simulink model "FOC_physical_2_Testing_mathmatical"  (R2024b)
settings: Solver=FixedStepAuto  StartTime=0.0  StopTime=4  FixedStep=1e-5  RelTol=1e-3
undefined symbols (not defined in the file): B, DiscIntNeverNeededParam, Down, dspblkCoreblockFVToolHelper, gcbh, GPTRIP1SEL, J, Ki_current, Ki_q, Ki_s, Ki_speed, Kp_current, Kp_q, Kp_s, Kp_speed, lambda, lamdaM, Ld, Ls, ma, P, Rs, T_max, T_period, Tc, TZ1, Up, Vdc
libraries: simulink x12, c2802xlib x7, spsIGBTDiodeLib x6, spsCurrentMeasurementLib x3, eeStairGenerator x2, spsStairGeneratorLib x2, spsDCVoltageSourceLib x1, spsPermanentMagnetSynchronousMachineLib x1, eeGeneralControl x1, mcbpositiondecoderlib x1, c280xlib x1, spspowerguiLib x1
(part 2 of 3)

== system FOC_physical_2_Testing_mathmatical/SVPWM Technique/Step 3- Determine the switching time of each transistor (S1 to S6)  ==
  T1 : Inport
  T2 : Inport  Port=2
  T0 : Inport  Port=3
  S : Inport  Port=4
  Fcn : Fcn  Expr=(T_period)-u(3)/2
  Fcn1 : Fcn  Expr=u(3)/2+u(2)
  Fcn2 : Fcn  Expr=u(3)/2
  Fcn3 : Fcn  Expr=u(3)/2+u(1)
  Mux1 : Mux  Inputs=3
  Sector detection1 : MATLAB Function  TreatAsAtomicUnit=on
  Ts1 : Outport
  Ts3 : Outport  Port=2
  Ts5 : Outport  Port=3
  wires:
  Sector detection1/1(Ts1) -> Ts1/1
  Sector detection1/3(Ts5) -> Ts5/1
  Sector detection1/2(Ts3) -> Ts3/1
  T0/1 -> Mux1/3
  T2/1 -> Mux1/2
  T1/1 -> Mux1/1
  Fcn2/1 -> Sector detection1/4(w)
  Fcn/1 -> Sector detection1/2(u)
  Fcn3/1 -> Sector detection1/5(g)
  Mux1/1 -> Fcn2/1, Fcn3/1, Fcn1/1, Fcn/1
  Fcn1/1 -> Sector detection1/3(v)
  S/1 -> Sector detection1/1(s)

== system FOC_physical_2_Testing_mathmatical/Subsystem/Forward Clacke ==
  Iu : Inport
  Iv : Inport  Port=2
  Iw : Inport  Port=3
  Gain : Gain  Gain=0.5
  Gain1 : Gain  Gain=0.5
  Gain2 : Gain  Gain=2/3
  Gain3 : Gain  Gain=sqrt(3)/2
  Gain4 : Gain  Gain=2/3
  Sum : Sum  Inputs=+--
  Sum1 : Sum  Inputs=+-
  I_alpha : Outport
  I_beta : Outport  Port=2
  wires:
  Iv/1 -> Gain/1, Sum1/1
  Gain/1 -> Sum/2
  Gain2/1 -> I_alpha/1
  Sum1/1 -> Gain3/1
  Gain1/1 -> Sum/3
  Iw/1 -> Gain1/1, Sum1/2
  Sum/1 -> Gain2/1
  Gain3/1 -> Gain4/1
  Iu/1 -> Sum/1
  Gain4/1 -> I_beta/1

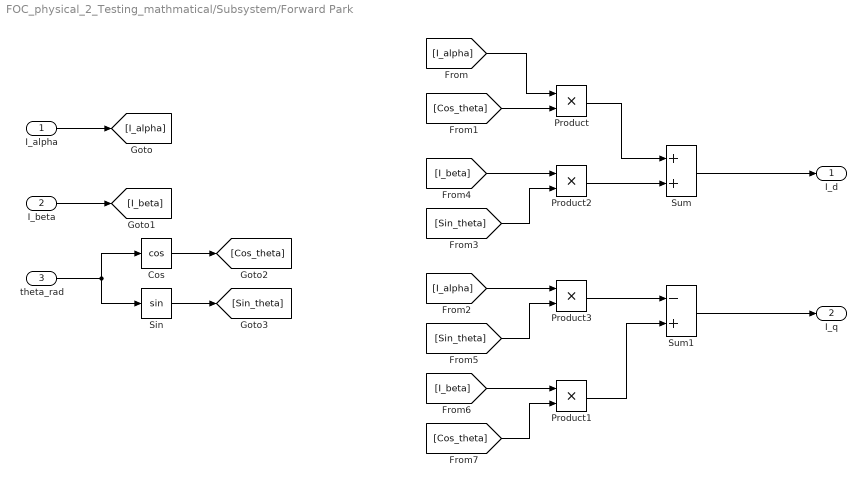
== system FOC_physical_2_Testing_mathmatical/Subsystem/Forward Park ==
  I_alpha : Inport
  I_beta : Inport  Port=2
  theta_rad : Inport  Port=3
  Cos : Trigonometry  Operator=cos
  Product{,1..3} (4 alike) : Product
  Sin : Trigonometry
  Sum : Sum
  Sum1 : Sum  Inputs=-+
  I_d : Outport
  I_q : Outport  Port=2
  wires:
  [Cos_theta] -> Product1/2
  [I_beta] -> Product1/1
  [Sin_theta] -> Product3/2
  [I_alpha] -> Product3/1
  Product1/1 -> Sum1/2
  [I_beta] -> Product2/1
  [Sin_theta] -> Product2/2
  [Cos_theta] -> Product/2
  Sin/1 -> [Sin_theta]
  Cos/1 -> [Cos_theta]
  theta_rad/1 -> Cos/1, Sin/1
  [I_alpha] -> Product/1
  I_beta/1 -> [I_beta]
  I_alpha/1 -> [I_alpha]
  Product3/1 -> Sum1/1
  Product2/1 -> Sum/2
  Product/1 -> Sum/1
  Sum1/1 -> I_q/1
  Sum/1 -> I_d/1

== system FOC_physical_2_Testing_mathmatical/Subsystem/Inverse Transformation ==
  Vq : Inport
  theta : Inport  Port=2
  Vd : Inport  Port=3
  "Inverse Park " : Subsystem  Commented=on
  dq to abc : Subsystem
  inverse Clark : Subsystem  Commented=on
  Va : Outport
  Vb : Outport  Port=2
  Vc : Outport  Port=3
  wires:
  theta/1 -> dq to abc/3(theta)
  Vq/1 -> dq to abc/1(V_q*)
  Vd/1 -> dq to abc/2(V_d*)
  dq to abc/1(Va*) -> Va/1
  dq to abc/2(Vb*) -> Vb/1
  dq to abc/3(Vc*) -> Vc/1

== system FOC_physical_2_Testing_mathmatical/Subsystem/SVPWM ==
  Va : Inport
  Vb : Inport  Port=2
  Vc : Inport  Port=3
  Vdc : Inport  Port=4
  Repeating Sequence : simulink/Sources/Repeating Sequence  rep_seq_t="[0 (T_period)/2  (T_period) ]"  rep_seq_y=[0 (T_period) 0]
  Scope : Scope  NumInputPorts=3
  Scope4 : Scope  NumInputPorts=4
  Sector detection : MATLAB Function  TreatAsAtomicUnit=on
  Subsystem : Subsystem
  Subsystem1 : Subsystem
  Subsystem2 : Subsystem
  Subsystem3 : Subsystem  Commented=on
  Subsystem4 : Subsystem  Commented=on
  Valpha and Vbeta Clark Trans : Subsystem
  TS1 : Outport
  TS3 : Outport  Port=2
  TS5 : Outport  Port=3
  wires:
  Valpha and Vbeta Clark Trans/1(Valpha) -> Subsystem/1(Valpha)
  Valpha and Vbeta Clark Trans/2(Vbeta) -> Subsystem/2(Vbeta)
  Vb/1 -> Scope/2, Valpha and Vbeta Clark Trans/2(Vb)
  Subsystem/2(angle) -> Sector detection/1(u), Subsystem1/2(angle)
  Vc/1 -> Scope/3, Valpha and Vbeta Clark Trans/3(Vc)
  Va/1 -> Valpha and Vbeta Clark Trans/1(Va), Scope/1
  Subsystem/1(Vref) -> Subsystem1/1(Vref)
  Sector detection/1(S) -> Subsystem1/3(Sector), Subsystem2/4(Sector definiton)  "Sector definiton"
  Subsystem1/2(T2) -> Scope4/2, Subsystem2/2(T2)
  Subsystem1/1(T1) -> Scope4/1, Subsystem2/1(T1)
  Subsystem1/3(T0) -> Subsystem2/3(T0), Scope4/3
  Subsystem2/2(TS3) -> TS3/1
  Subsystem2/1(TS1) -> TS1/1
  Subsystem2/3(TS5) -> TS5/1
  Vdc/1 -> Subsystem1/4(Vdc)

== system FOC_physical_2_Testing_mathmatical/Subsystem/Speed PI Controller with anti-windup ==
  Mech Speed ref : Inport
  Speed act : Inport  Port=2
  " max current" : Saturate  UpperLimit=T_max/((3/2)*lamdaM*P)  LowerLimit=0
  Abs : Abs  SaturateOnIntegerOverflow=off
  Abs1 : Abs  SaturateOnIntegerOverflow=off
  Compare To Constant1 : simulink/Logic and Bit Operations/Compare To Constant  relop=<=  const=1e-4  OutDataTypeStr=boolean
  Integrator2 : Integrator  ExternalReset=falling
  "Ki " : Gain  Gain=Ki_speed
  Kp : Gain  Gain=Kp_speed
  Product : Product  Inputs=3
  Scope : Scope
  Scope1 : Scope  NumInputPorts=2
  Scope2 : Scope  NumInputPorts=2
  Scope3 : Scope  NumInputPorts=3
  Scope4 : Scope  NumInputPorts=2
  Sum : Sum  Inputs=|+-
  Sum1 : Sum
  Sum2 : Sum  Inputs=|-+
  rpm_to_rad/s : Gain  Gain=pi/30
  stop integration at low speed : Relay  OnSwitchValue=100  OffSwitchValue=-100
  I_q* : Outport
  wires:
  " max current"/1 -> Scope2/1, Sum2/1, I_q*/1
  Sum/1 -> rpm_to_rad/s/1
  rpm_to_rad/s/1 -> Kp/1, Scope3/1, "Ki "/1
  stop integration at low speed/1 -> Integrator2/2, Product/3, Scope4/1
  Abs1/1 -> Scope4/2, stop integration at low speed/1
  Compare To Constant1/1 -> Scope/1, Product/1
  Abs/1 -> Compare To Constant1/1
  Sum2/1 -> Abs/1
  Sum1/1 -> " max current"/1, Sum2/2, Scope3/3, Scope2/2
  Integrator2/1 -> Sum1/2, Scope1/2
  Product/1 -> Integrator2/1, Scope1/1
  "Ki "/1 -> Product/2
  Kp/1 -> Sum1/1, Scope3/2
  Speed act/1 -> Sum/2, Abs1/1
  Mech Speed ref/1 -> Sum/1

== system FOC_physical_2_Testing_mathmatical/Subsystem/Subsystem ==
  Va : Inport
  Vb : Inport  Port=2
  Vc : Inport  Port=3
  TL : Inport  Port=4
  Current Calculation1 : Subsystem
  Display : Display
  Display1 : Display
  Display2 : Display
  Gain2 : Gain  Gain=60/(2*pi)
  Gain3 : Gain  Gain=1/P
  Park and Clark transformation1 : Subsystem
  Scope : Scope  NumInputPorts=2
  Speed1 : Subsystem
  Torque 1 : Subsystem
  Te : Outport
  Wm : Outport  Port=2
  Id : Outport  Port=3
  Iq : Outport  Port=4
  Theta : Outport  Port=5
  wires:
  [Wr] -> Current Calculation1/3(wr)
  Va/1 -> Display2/1, Park and Clark transformation1/1(Va)
  Park and Clark transformation1/2(Vq) -> Current Calculation1/2(Vq), Display1/1
  Torque 1/1(Te) -> Scope/2, Te/1, Speed1/1(Te)
  Speed1/1(wr) -> Gain2/1, [Wr]
  Park and Clark transformation1/1(Vd) -> Display/1, Current Calculation1/1(Vd)
  Gain2/1 -> Gain3/1
  Speed1/2(Theta) -> Park and Clark transformation1/4(Theta), Theta/1
  Current Calculation1/2(Iq) -> Torque 1/2(Iq), Iq/1
  Current Calculation1/1(Id) -> Id/1, Torque 1/1(Id)
  Vb/1 -> Park and Clark transformation1/2(Vb)
  Gain3/1 -> Scope/1, Wm/1  "N_actual"
  Vc/1 -> Park and Clark transformation1/3(Vc)
  TL/1 -> Speed1/2(TL)

== system FOC_physical_2_Testing_mathmatical/Subsystem/Voltage Decoupling  ==
  V_q* : Inport
  V_d* : Inport  Port=2
  Gain : Gain  Gain=2*pi/60
  Gain1 : Gain  Gain=P
  Gain2 : Gain  Gain=P
  Gain3 : Gain  Gain=P
  Gain4 : Gain  Gain=2*pi/60
  Gain5 : Gain  Gain=2*pi/60
  Lambda_m : Constant  Value=lamdaM
  Lambda_m1 : Constant  Value=Ls
  Ld : Constant  Value=Ls
  Product : Product  Inputs=3
  Product1 : Product
  Product2 : Product  Inputs=3
  Sum3 : Sum  Inputs=+++
  Sum4 : Sum  Inputs=|+-
  Vq : Outport
  Vd : Outport  Port=2
  wires:
  [Id] -> Product/1
  V_q*/1 -> Sum3/2
  Gain1/1 -> Product2/2
  Product2/1 -> Sum4/2
  [Iq] -> Product2/1
  Product1/1 -> Sum3/3
  [W_act] -> Gain5/1
  Gain2/1 -> Product/2
  [W_act] -> Gain/1
  Ld/1 -> Product/3
  [W_act] -> Gain4/1
  Product/1 -> Sum3/1
  Gain3/1 -> Product1/1
  Lambda_m/1 -> Product1/2
  Lambda_m1/1 -> Product2/3
  Sum3/1 -> Vq/1
  V_d*/1 -> Sum4/1
  Sum4/1 -> Vd/1
  Gain/1 -> Gain2/1
  Gain4/1 -> Gain3/1
  Gain5/1 -> Gain1/1

== system FOC_physical_2_Testing_mathmatical/Subsystem/d-current PI controller with anti-windup ==
  Id command : Inport
  Id act : Inport  Port=2
  Integrator2 : Integrator
  "Ki " : Gain  Gain=Ki_current
  Kp : Gain  Gain=Kp_current
  Product : Product
  Scope : Scope
  Scope1 : Scope  NumInputPorts=2
  Scope2 : Scope  NumInputPorts=2
  Scope3 : Scope  NumInputPorts=3
  Sum : Sum  Inputs=|+-
  Sum1 : Sum
  V_d* : Outport
  wires:
  Sum1/1 -> V_d*/1, Scope3/3, Scope2/2
  Integrator2/1 -> Sum1/2, Scope1/2
  Product/1 -> Integrator2/1, Scope1/1
  "Ki "/1 -> Product/2
  Kp/1 -> Sum1/1, Scope3/2
  Sum/1 -> Kp/1, Scope3/1, "Ki "/1
  Id act/1 -> Sum/2
  Id command/1 -> Sum/1
  [stop_d_integrator] -> Product/1, Scope/1

== system FOC_physical_2_Testing_mathmatical/Subsystem/q-current PI controller with anti-windup ==
  Iq command : Inport
  Iq act : Inport  Port=2
  Integrator2 : Integrator
  "Ki " : Gain  Gain=Ki_current
  Kp : Gain  Gain=Kp_current
  Product : Product
  Scope : Scope
  Scope1 : Scope  NumInputPorts=2
  Scope2 : Scope  NumInputPorts=2
  Scope3 : Scope  NumInputPorts=3
  Sum : Sum  Inputs=|+-
  Sum1 : Sum
  V_q* : Outport
  wires:
  Iq command/1 -> Sum/1
  Iq act/1 -> Sum/2
  Sum/1 -> "Ki "/1, Scope3/1, Kp/1
  Kp/1 -> Scope3/2, Sum1/1
  "Ki "/1 -> Product/2
  Product/1 -> Integrator2/1, Scope1/1
  Integrator2/1 -> Scope1/2, Sum1/2
  Sum1/1 -> V_q*/1, Scope2/2, Scope3/3
  [stop_q_integrator] -> Scope/1, Product/1

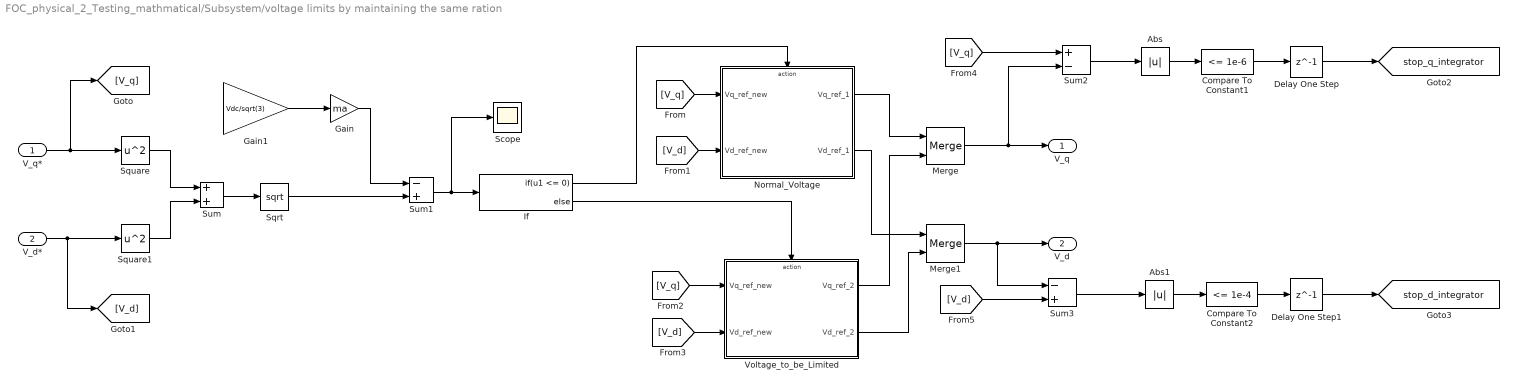
== system FOC_physical_2_Testing_mathmatical/Subsystem/voltage limits by maintaining the same ration ==
  V_q* : Inport
  V_d* : Inport  Port=2
  Abs : Abs  SaturateOnIntegerOverflow=off
  Abs1 : Abs  SaturateOnIntegerOverflow=off
  Compare To Constant1 : simulink/Logic and Bit Operations/Compare To Constant  relop=<=  const=1e-6  OutDataTypeStr=boolean
  Compare To Constant2 : simulink/Logic and Bit Operations/Compare To Constant  relop=<=  const=1e-4  OutDataTypeStr=boolean
  Delay One Step : Delay  DelayLength=1
  Delay One Step1 : Delay  DelayLength=1
  Gain : Gain  Gain=ma
  Gain1 : Gain  Gain=Vdc/sqrt(3)
  If : If  IfExpression=u1 <= 0
  Merge : Merge
  Merge1 : Merge
  Normal_Voltage : Subsystem  TreatAsAtomicUnit=on
      settings: RTWSystemCode=Inline  RTWFcnNameOpts=Use subsystem name  RTWFileNameOpts=Use subsystem name
  Scope : Scope
  Sqrt : Sqrt
  Square : Math  Operator=square
  Square1 : Math  Operator=square
  Sum : Sum
  Sum1 : Sum  Inputs=-+
  Sum2 : Sum  Inputs=+-
  Sum3 : Sum  Inputs=-+
  Voltage_to_be_Limited : Subsystem  TreatAsAtomicUnit=on
      settings: RTWSystemCode=Inline  RTWFcnNameOpts=Use subsystem name  RTWFileNameOpts=Use subsystem name
  V_q : Outport
  V_d : Outport  Port=2
  tag scope: stop_d_integrator=global, stop_q_integrator=global
  wires:
  V_q*/1 -> [V_q], Square/1
  V_d*/1 -> [V_d], Square1/1
  Sum/1 -> Sqrt/1
  Square/1 -> Sum/1
  Square1/1 -> Sum/2
  Sqrt/1 -> Sum1/2
  Merge/1 -> Sum2/2, V_q/1
  Gain/1 -> Sum1/1
  Sum1/1 -> Scope/1, If/1
  If/1 -> Normal_Voltage/Action
  [V_q] -> Normal_Voltage/1(Vq_ref_new)
  [V_d] -> Normal_Voltage/2(Vd_ref_new)
  If/2 -> Voltage_to_be_Limited/Action
  Voltage_to_be_Limited/1(Vq_ref_2) -> Merge/2
  Normal_Voltage/1(Vq_ref_1) -> Merge/1
  Voltage_to_be_Limited/2(Vd_ref_2) -> Merge1/2
  Normal_Voltage/2(Vd_ref_1) -> Merge1/1
  [V_q] -> Voltage_to_be_Limited/1(Vq_ref_new)
  [V_d] -> Voltage_to_be_Limited/2(Vd_ref_new)
  [V_q] -> Sum2/1
  Merge1/1 -> Sum3/1, V_d/1
  [V_d] -> Sum3/2
  Delay One Step/1 -> [stop_q_integrator]
  Delay One Step1/1 -> [stop_d_integrator]
  Abs/1 -> Compare To Constant1/1
  Compare To Constant1/1 -> Delay One Step/1
  Sum2/1 -> Abs/1
  Sum3/1 -> Abs1/1
  Abs1/1 -> Compare To Constant2/1
  Compare To Constant2/1 -> Delay One Step1/1
  Gain1/1 -> Gain/1

== system FOC_physical_2_Testing_mathmatical/Subsystem3/Forward Clacke ==
  Iu : Inport
  Iv : Inport  Port=2
  Iw : Inport  Port=3
  Gain : Gain  Gain=0.5
  Gain1 : Gain  Gain=0.5
  Gain2 : Gain  Gain=2/3
  Gain3 : Gain  Gain=sqrt(3)/2
  Gain4 : Gain  Gain=2/3
  Sum : Sum  Inputs=+--
  Sum1 : Sum  Inputs=+-
  I_alpha : Outport
  I_beta : Outport  Port=2
  wires:
  Iv/1 -> Gain/1, Sum1/1
  Gain/1 -> Sum/2
  Gain2/1 -> I_alpha/1
  Sum1/1 -> Gain3/1
  Gain1/1 -> Sum/3
  Iw/1 -> Gain1/1, Sum1/2
  Sum/1 -> Gain2/1
  Gain3/1 -> Gain4/1
  Iu/1 -> Sum/1
  Gain4/1 -> I_beta/1

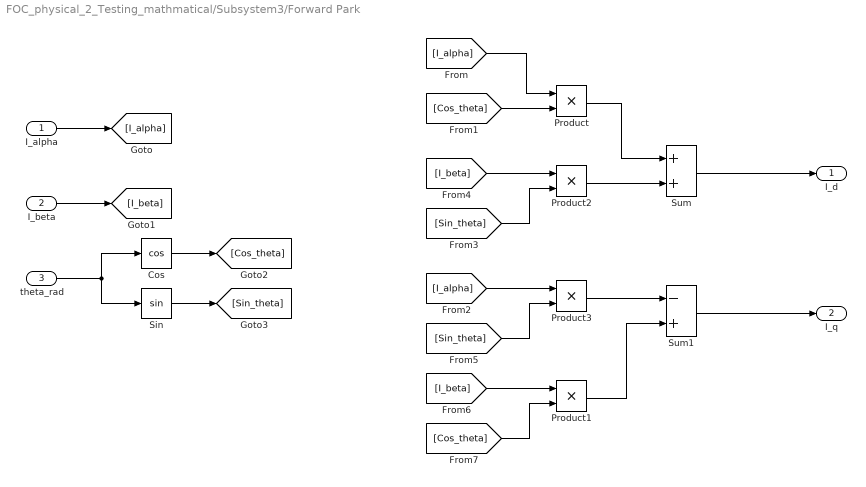
== system FOC_physical_2_Testing_mathmatical/Subsystem3/Forward Park ==
  I_alpha : Inport
  I_beta : Inport  Port=2
  theta_rad : Inport  Port=3
  Cos : Trigonometry  Operator=cos
  Product{,1..3} (4 alike) : Product
  Sin : Trigonometry
  Sum : Sum
  Sum1 : Sum  Inputs=-+
  I_d : Outport
  I_q : Outport  Port=2
  wires:
  [Cos_theta] -> Product1/2
  [I_beta] -> Product1/1
  [Sin_theta] -> Product3/2
  [I_alpha] -> Product3/1
  Product1/1 -> Sum1/2
  [I_beta] -> Product2/1
  [Sin_theta] -> Product2/2
  [Cos_theta] -> Product/2
  Sin/1 -> [Sin_theta]
  Cos/1 -> [Cos_theta]
  theta_rad/1 -> Cos/1, Sin/1
  [I_alpha] -> Product/1
  I_beta/1 -> [I_beta]
  I_alpha/1 -> [I_alpha]
  Product3/1 -> Sum1/1
  Product2/1 -> Sum/2
  Product/1 -> Sum/1
  Sum1/1 -> I_q/1
  Sum/1 -> I_d/1

== system FOC_physical_2_Testing_mathmatical/Subsystem3/Inverse Transformation ==
  Vq : Inport
  theta : Inport  Port=2
  Vd : Inport  Port=3
  "Inverse Park " : Subsystem  Commented=on
  dq to abc : Subsystem
  inverse Clark : Subsystem  Commented=on
  Va : Outport
  Vb : Outport  Port=2
  Vc : Outport  Port=3
  wires:
  theta/1 -> dq to abc/3(theta)
  Vq/1 -> dq to abc/1(V_q*)
  Vd/1 -> dq to abc/2(V_d*)
  dq to abc/1(Va*) -> Va/1
  dq to abc/2(Vb*) -> Vb/1
  dq to abc/3(Vc*) -> Vc/1

== system FOC_physical_2_Testing_mathmatical/Subsystem3/SVPWM ==
  Va : Inport
  Vb : Inport  Port=2
  Vc : Inport  Port=3
  Vdc : Inport  Port=4
  Scope : Scope  NumInputPorts=3
  Scope4 : Scope  NumInputPorts=4
  Sector detection : MATLAB Function  TreatAsAtomicUnit=on
  Subsystem : Subsystem
  Subsystem1 : Subsystem
  Subsystem2 : Subsystem
  Subsystem3 : Subsystem  Commented=on
  Subsystem4 : Subsystem  Commented=on
  Valpha and Vbeta Clark Trans : Subsystem
  TS1 : Outport
  TS3 : Outport  Port=2
  TS5 : Outport  Port=3
  wires:
  Valpha and Vbeta Clark Trans/1(Valpha) -> Subsystem/1(Valpha)
  Valpha and Vbeta Clark Trans/2(Vbeta) -> Subsystem/2(Vbeta)
  Vb/1 -> Scope/2, Valpha and Vbeta Clark Trans/2(Vb)
  Subsystem/2(angle) -> Sector detection/1(u), Subsystem1/2(angle)
  Vc/1 -> Scope/3, Valpha and Vbeta Clark Trans/3(Vc)
  Va/1 -> Valpha and Vbeta Clark Trans/1(Va), Scope/1
  Subsystem/1(Vref) -> Subsystem1/1(Vref)
  Sector detection/1(S) -> Subsystem1/3(Sector), Subsystem2/4(Sector definiton)  "Sector definiton"
  Subsystem1/2(T2) -> Scope4/2, Subsystem2/2(T2)
  Subsystem1/1(T1) -> Scope4/1, Subsystem2/1(T1)
  Subsystem1/3(T0) -> Subsystem2/3(T0), Scope4/3
  Subsystem2/2(TS3) -> TS3/1
  Subsystem2/1(TS1) -> TS1/1
  Subsystem2/3(TS5) -> TS5/1
  Vdc/1 -> Subsystem1/4(Vdc)

== system FOC_physical_2_Testing_mathmatical/Subsystem3/Speed PI Controller with anti-windup ==
  Mech Speed ref : Inport
  Speed act : Inport  Port=2
  " max current" : Saturate  UpperLimit=T_max/((3/2)*lamdaM*P)  LowerLimit=-T_max/((3/2)*lamdaM*P)
  Abs : Abs  SaturateOnIntegerOverflow=off
  Abs1 : Abs  SaturateOnIntegerOverflow=off
  Compare To Constant1 : simulink/Logic and Bit Operations/Compare To Constant  relop=<=  const=1e-4  OutDataTypeStr=boolean
  Discrete-Time Integrator : DiscreteIntegrator  ExternalReset=falling  SampleTime=-1  ICPrevOutput=DiscIntNeverNeededParam  ICPrevScaledInput=DiscIntNeverNeededParam
  "Ki " : Gain  Gain=Ki_speed
  Kp : Gain  Gain=Kp_speed
  Product : Product  Inputs=3
  Scope : Scope
  Scope1 : Scope  NumInputPorts=2
  Scope2 : Scope  NumInputPorts=2
  Scope3 : Scope  NumInputPorts=3
  Scope4 : Scope  NumInputPorts=2
  Sum : Sum  Inputs=|+-
  Sum1 : Sum
  Sum2 : Sum  Inputs=|-+
  rpm_to_rad/s : Gain  Gain=pi/30
  stop integration at low speed : Relay  OnSwitchValue=100  OffSwitchValue=-100  OutDataTypeStr=boolean
  I_q* : Outport
  wires:
  " max current"/1 -> Scope2/1, Sum2/1, I_q*/1
  Sum/1 -> rpm_to_rad/s/1
  rpm_to_rad/s/1 -> Kp/1, Scope3/1, "Ki "/1
  Abs1/1 -> Scope4/2, stop integration at low speed/1
  Compare To Constant1/1 -> Scope/1, Product/1
  Abs/1 -> Compare To Constant1/1
  Sum2/1 -> Abs/1
  Sum1/1 -> " max current"/1, Sum2/2, Scope3/3, Scope2/2
  Discrete-Time Integrator/1 -> Sum1/2, Scope1/2
  Product/1 -> Discrete-Time Integrator/1, Scope1/1
  "Ki "/1 -> Product/2
  Kp/1 -> Sum1/1, Scope3/2
  Speed act/1 -> Sum/2, Abs1/1
  Mech Speed ref/1 -> Sum/1
  stop integration at low speed/1 -> Discrete-Time Integrator/2, Product/3, Scope4/1

== system FOC_physical_2_Testing_mathmatical/Subsystem3/Subsystem ==
  Va : Inport
  Vb : Inport  Port=2
  Vc : Inport  Port=3
  TL : Inport  Port=4
  Current Calculation1 : Subsystem
  Display : Display
  Display1 : Display
  Display2 : Display
  Gain2 : Gain  Gain=60/(2*pi)
  Gain3 : Gain  Gain=1/P
  Park and Clark transformation1 : Subsystem
  Scope : Scope  NumInputPorts=2
  Speed1 : Subsystem
  Torque 1 : Subsystem
  Te : Outport
  Wm : Outport  Port=2
  Id : Outport  Port=3
  Iq : Outport  Port=4
  Theta : Outport  Port=5
  wires:
  [Wr] -> Current Calculation1/3(wr)
  Va/1 -> Display2/1, Park and Clark transformation1/1(Va)
  Park and Clark transformation1/2(Vq) -> Current Calculation1/2(Vq), Display1/1
  Torque 1/1(Te) -> Scope/2, Te/1, Speed1/1(Te)
  Speed1/1(wr) -> Gain2/1, [Wr]
  Park and Clark transformation1/1(Vd) -> Display/1, Current Calculation1/1(Vd)
  Gain2/1 -> Gain3/1
  Speed1/2(Theta) -> Park and Clark transformation1/4(Theta), Theta/1
  Current Calculation1/2(Iq) -> Torque 1/2(Iq), Iq/1
  Current Calculation1/1(Id) -> Id/1, Torque 1/1(Id)
  Vb/1 -> Park and Clark transformation1/2(Vb)
  Gain3/1 -> Scope/1, Wm/1  "N_actual"
  Vc/1 -> Park and Clark transformation1/3(Vc)
  TL/1 -> Speed1/2(TL)

== system FOC_physical_2_Testing_mathmatical/Subsystem3/Voltage Decoupling  ==
  V_q* : Inport
  V_d* : Inport  Port=2
  Gain1 : Gain  Gain=P
  Gain2 : Gain  Gain=P
  Gain3 : Gain  Gain=P
  Lambda_m : Constant  Value=lamdaM
  Lambda_m1 : Constant  Value=lamdaM
  Ld : Constant  Value=Ls
  Product : Product  Inputs=3
  Product1 : Product
  Product2 : Product  Inputs=3
  Sum3 : Sum  Inputs=+++
  Sum4 : Sum  Inputs=|+-
  Out1 : Outport
  Out2 : Outport  Port=2
  wires:
  [Id] -> Product/1
  V_q*/1 -> Sum3/2
  Gain1/1 -> Product2/2
  Product2/1 -> Sum4/2
  [Iq] -> Product2/1
  Product1/1 -> Sum3/3
  [W_act] -> Gain1/1
  Gain2/1 -> Product/2
  [W_act] -> Gain2/1
  Ld/1 -> Product/3
  [W_act] -> Gain3/1
  Product/1 -> Sum3/1
  Gain3/1 -> Product1/1
  Lambda_m/1 -> Product1/2
  Lambda_m1/1 -> Product2/3
  Sum3/1 -> Out1/1
  V_d*/1 -> Sum4/1
  Sum4/1 -> Out2/1

== system FOC_physical_2_Testing_mathmatical/Subsystem3/d-current PI controller with anti-windup ==
  Id command : Inport
  Id act : Inport  Port=2
  Discrete-Time Integrator : DiscreteIntegrator  SampleTime=-1  ICPrevOutput=DiscIntNeverNeededParam  ICPrevScaledInput=DiscIntNeverNeededParam
  "Ki " : Gain  Gain=Ki_current
  Kp : Gain  Gain=Kp_current
  Product : Product
  Scope : Scope
  Scope1 : Scope  NumInputPorts=2
  Scope2 : Scope  NumInputPorts=2
  Scope3 : Scope  NumInputPorts=3
  Sum : Sum  Inputs=|+-
  Sum1 : Sum
  V_d* : Outport
  wires:
  Sum1/1 -> V_d*/1, Scope3/3, Scope2/2
  Discrete-Time Integrator/1 -> Sum1/2, Scope1/2
  Product/1 -> Discrete-Time Integrator/1, Scope1/1
  "Ki "/1 -> Product/2
  Kp/1 -> Sum1/1, Scope3/2
  Sum/1 -> Kp/1, Scope3/1, "Ki "/1
  Id act/1 -> Sum/2
  Id command/1 -> Sum/1
  [stop_d_integrator] -> Product/1, Scope/1

== system FOC_physical_2_Testing_mathmatical/Subsystem3/q-current PI controller with anti-windup ==
  Iq command : Inport
  Iq act : Inport  Port=2
  Discrete-Time Integrator : DiscreteIntegrator  SampleTime=-1  ICPrevOutput=DiscIntNeverNeededParam  ICPrevScaledInput=DiscIntNeverNeededParam
  "Ki " : Gain  Gain=Ki_current
  Kp : Gain  Gain=Kp_current
  Product : Product
  Scope : Scope
  Scope1 : Scope  NumInputPorts=2
  Scope2 : Scope  NumInputPorts=2
  Scope3 : Scope  NumInputPorts=3
  Sum : Sum  Inputs=|+-
  Sum1 : Sum
  V_q* : Outport
  wires:
  Iq command/1 -> Sum/1
  Iq act/1 -> Sum/2
  Sum/1 -> "Ki "/1, Scope3/1, Kp/1
  Kp/1 -> Scope3/2, Sum1/1
  "Ki "/1 -> Product/2
  Product/1 -> Discrete-Time Integrator/1, Scope1/1
  Discrete-Time Integrator/1 -> Scope1/2, Sum1/2
  Sum1/1 -> V_q*/1, Scope2/2, Scope3/3
  [stop_q_integrator] -> Scope/1, Product/1

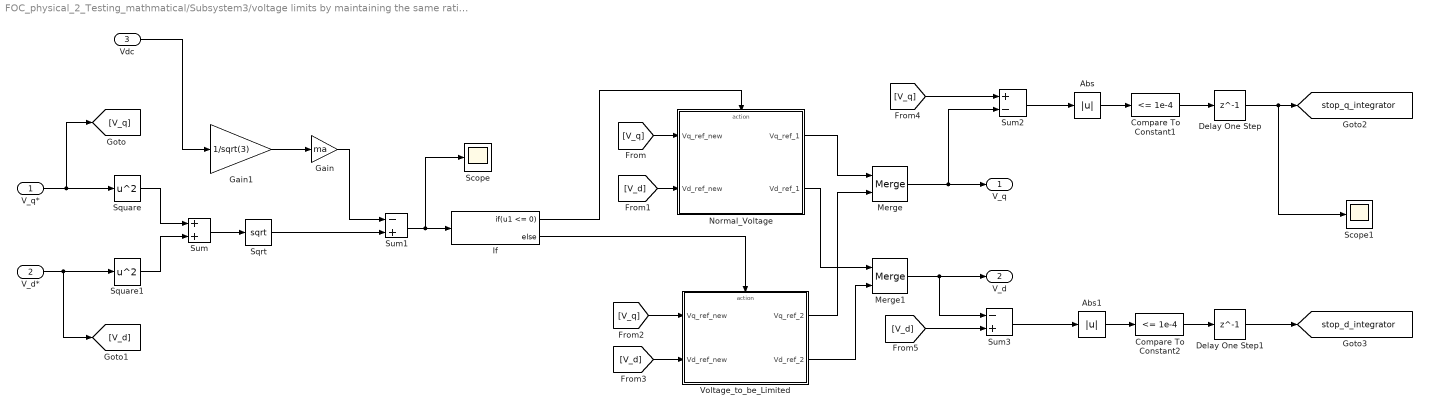
== system FOC_physical_2_Testing_mathmatical/Subsystem3/voltage limits by maintaining the same ration ==
  V_q* : Inport
  V_d* : Inport  Port=2
  Vdc : Inport  Port=3
  Abs : Abs  SaturateOnIntegerOverflow=off
  Abs1 : Abs  SaturateOnIntegerOverflow=off
  Compare To Constant1 : simulink/Logic and Bit Operations/Compare To Constant  relop=<=  const=1e-4  OutDataTypeStr=boolean
  Compare To Constant2 : simulink/Logic and Bit Operations/Compare To Constant  relop=<=  const=1e-4  OutDataTypeStr=boolean
  Delay One Step : Delay  DelayLength=1
  Delay One Step1 : Delay  DelayLength=1
  Gain : Gain  Gain=ma  OutDataTypeStr=Inherit: Same as input  ParamDataTypeStr=Inherit: Same as input
  Gain1 : Gain  Gain=1/sqrt(3)
  If : If  IfExpression=u1 <= 0
  Merge : Merge
  Merge1 : Merge
  Normal_Voltage : Subsystem  TreatAsAtomicUnit=on
      settings: RTWSystemCode=Inline  RTWFcnNameOpts=Use subsystem name  RTWFileNameOpts=Use subsystem name
  Scope : Scope
  Scope1 : Scope
  Sqrt : Sqrt
  Square : Math  Operator=square
  Square1 : Math  Operator=square
  Sum : Sum
  Sum1 : Sum  Inputs=-+
  Sum2 : Sum  Inputs=+-
  Sum3 : Sum  Inputs=-+
  Voltage_to_be_Limited : Subsystem  TreatAsAtomicUnit=on
      settings: RTWSystemCode=Inline  RTWFcnNameOpts=Use subsystem name  RTWFileNameOpts=Use subsystem name
  V_q : Outport
  V_d : Outport  Port=2
  tag scope: stop_d_integrator=global, stop_q_integrator=global
  wires:
  V_q*/1 -> [V_q], Square/1
  V_d*/1 -> [V_d], Square1/1
  Sum/1 -> Sqrt/1
  Square/1 -> Sum/1
  Square1/1 -> Sum/2
  Sqrt/1 -> Sum1/2
  Merge/1 -> Sum2/2, V_q/1
  Gain/1 -> Sum1/1
  Sum1/1 -> Scope/1, If/1
  If/1 -> Normal_Voltage/Action
  [V_q] -> Normal_Voltage/1(Vq_ref_new)
  [V_d] -> Normal_Voltage/2(Vd_ref_new)
  If/2 -> Voltage_to_be_Limited/Action
  Voltage_to_be_Limited/1(Vq_ref_2) -> Merge/2
  Normal_Voltage/1(Vq_ref_1) -> Merge/1
  Voltage_to_be_Limited/2(Vd_ref_2) -> Merge1/2
  Normal_Voltage/2(Vd_ref_1) -> Merge1/1
  [V_q] -> Voltage_to_be_Limited/1(Vq_ref_new)
  [V_d] -> Voltage_to_be_Limited/2(Vd_ref_new)
  [V_q] -> Sum2/1
  Merge1/1 -> Sum3/1, V_d/1
  [V_d] -> Sum3/2
  Delay One Step1/1 -> [stop_d_integrator]
  Abs/1 -> Compare To Constant1/1
  Compare To Constant1/1 -> Delay One Step/1
  Sum2/1 -> Abs/1
  Sum3/1 -> Abs1/1
  Abs1/1 -> Compare To Constant2/1
  Compare To Constant2/1 -> Delay One Step1/1
  Vdc/1 -> Gain1/1
  Gain1/1 -> Gain/1
  Delay One Step/1 -> Scope1/1, [stop_q_integrator]

== system FOC_physical_2_Testing_mathmatical/Voltage limits/If Action Subsystem ==
  In3 : Inport
  In4 : Inport  Port=2
  Action Port : ActionPort  ActionPortLabel=if(u1 <= 0)
  Cast To Single : DataTypeConversion  OutDataTypeStr=single  SaturateOnIntegerOverflow=off  RndMeth=Floor
  Cast To Single1 : DataTypeConversion  OutDataTypeStr=single  SaturateOnIntegerOverflow=off  RndMeth=Floor
  Out2 : Outport
  Out3 : Outport  Port=2
  wires:
  In3/1 -> Cast To Single/1
  In4/1 -> Cast To Single1/1
  Cast To Single/1 -> Out2/1
  Cast To Single1/1 -> Out3/1

== system FOC_physical_2_Testing_mathmatical/Voltage limits/If Action Subsystem1 ==
  In3 : Inport
  In4 : Inport  Port=2
  Action Port : ActionPort  ActionPortLabel=else
  Divide1 : Product  Inputs=*/  OutDataTypeStr=single
  Divide2 : Product  Inputs=/*  OutDataTypeStr=single
  Gain : Gain  Gain=sqrt(3)
  Gain1 : Gain  Gain=325 * .95
  Gain2 : Gain  Gain=325 * .95
  Square : Math  Operator=square  OutDataTypeStr=single
  Square Root : Sqrt  OutDataTypeStr=single  IntermediateResultsDataTypeStr=single
  Square1 : Math  Operator=square  OutDataTypeStr=single
  Sum : Sum  OutDataTypeStr=single  AccumDataTypeStr=single
  Out2 : Outport
  Out3 : Outport  Port=2
  wires:
  Divide1/1 -> Out2/1
  Divide2/1 -> Out3/1
  Square/1 -> Sum/1
  In3/1 -> Gain1/1, Square/1
  Sum/1 -> Square Root/1
  Gain2/1 -> Divide2/2
  Gain/1 -> Divide2/1, Divide1/2
  Gain1/1 -> Divide1/1
  Square1/1 -> Sum/2
  Square Root/1 -> Gain/1
  In4/1 -> Square1/1, Gain2/1

== system FOC_physical_2_Testing_mathmatical/SVPWM Technique/Step 1- Determine Vd, Vq, Vref, and angle/Polar form ==
  In1 : Inport
  In2 : Inport  Port=2
  Add : Sum
  Atan2 : Trigonometry  Operator=atan2
  Sqrt : Sqrt
  Square : Math  Operator=square
  Square1 : Math  Operator=square
  V ref : Outport
  angle : Outport  Port=2
  wires:
  In1/1 -> Square/1, Atan2/2
  Add/1 -> Sqrt/1
  Sqrt/1 -> V ref/1
  In2/1 -> Square1/1, Atan2/1
  Atan2/1 -> angle/1
  Square/1 -> Add/1
  Square1/1 -> Add/2

== system FOC_physical_2_Testing_mathmatical/SVPWM Technique/Step 1- Determine Vd, Vq, Vref, and angle/Power variant Clark transformation  ==
  Va : Inport
  Vb : Inport  Port=2
  Vc : Inport  Port=3
  Gain : Gain  Gain=0.5
  Gain1 : Gain  Gain=0.5
  Gain2 : Gain  Gain=2/3
  Gain3 : Gain  Gain=sqrt(3)/2
  Gain4 : Gain  Gain=2/3
  Sum : Sum  Inputs=+--
  Sum1 : Sum  Inputs=+-
  V alpha : Outport
  V beta : Outport  Port=2
  wires:
  Gain4/1 -> V beta/1
  Gain2/1 -> V alpha/1
  Vb/1 -> Gain/1, Sum1/1
  Gain/1 -> Sum/2
  Sum1/1 -> Gain3/1
  Gain1/1 -> Sum/3
  Vc/1 -> Gain1/1, Sum1/2
  Sum/1 -> Gain2/1
  Gain3/1 -> Gain4/1
  Va/1 -> Sum/1

== system FOC_physical_2_Testing_mathmatical/SVPWM Technique/Step 2- Determine time duration T1, T2, T/angle_d ==
  angle : Inport
  Sector : Inport  Port=2
  Constant3 : Constant
  Gain : Gain  Gain=pi/3
  Subtract4 : Sum  Inputs=-+
  Subtract5 : Sum  Inputs=+-
  angle_d(0 - pi/3) : Outport
  wires:
  Gain/1 -> Subtract4/1
  Subtract5/1 -> Gain/1
  Constant3/1 -> Subtract5/2
  Subtract4/1 -> angle_d(0 - pi/3)/1
  Sector/1 -> Subtract5/1
  angle/1 -> Subtract4/2

== system FOC_physical_2_Testing_mathmatical/Subsystem/Inverse Transformation/Inverse Park  ==
  In1 : Inport
  In2 : Inport  Port=2
  In3 : Inport  Port=3
  Cos : Trigonometry  Operator=cos
  Cos1 : Trigonometry  Operator=cos
  Product{,1..3} (4 alike) : Product
  Sin : Trigonometry
  Sin1 : Trigonometry
  Subtract : Sum  Inputs=+-
  Subtract2 : Sum
  Valpha : Outport
  Vbeta : Outport  Port=2
  wires:
  Product3/1 -> Subtract2/1
  In3/1 -> Product2/2, Product1/2
  In1/1 -> Cos/1, [theta], Sin/1
  Subtract/1 -> Valpha/1  "Valpha"
  Product/1 -> Subtract/1
  Subtract2/1 -> Vbeta/1  "Vbeta"
  Product2/1 -> Subtract2/2
  Cos/1 -> Product/1
  Product1/1 -> Subtract/2
  [theta] -> Cos1/1
  In2/1 -> Product/2, Product3/1
  [theta] -> Sin1/1
  Sin/1 -> Product1/1
  Cos1/1 -> Product2/1
  Sin1/1 -> Product3/2

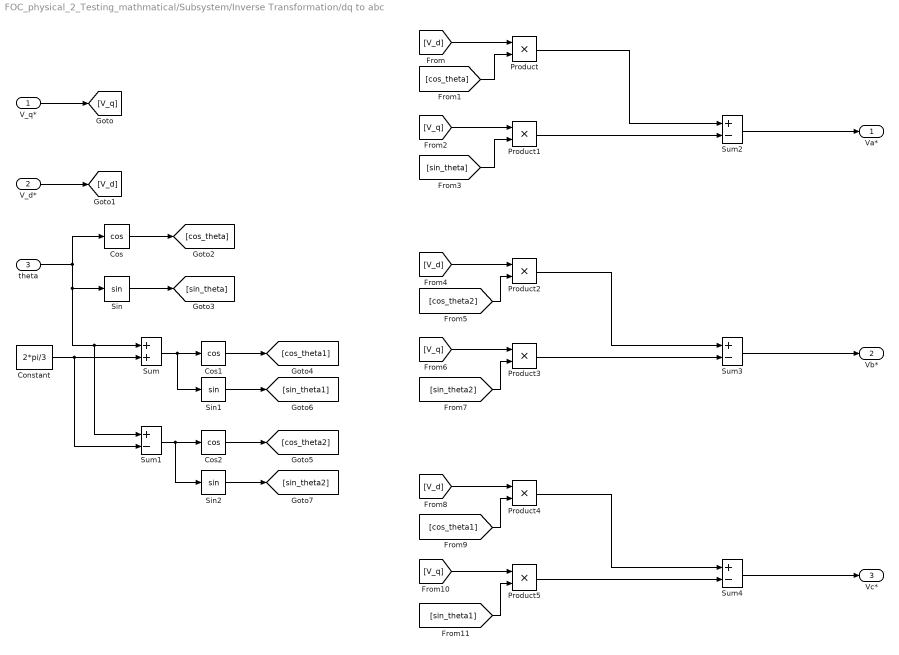
== system FOC_physical_2_Testing_mathmatical/Subsystem/Inverse Transformation/dq to abc ==
  V_q* : Inport
  V_d* : Inport  Port=2
  theta : Inport  Port=3
  Constant : Constant  Value=2*pi/3
  Cos : Trigonometry  Operator=cos
  Cos1 : Trigonometry  Operator=cos
  Cos2 : Trigonometry  Operator=cos
  Product{,1..5} (6 alike) : Product
  Sin : Trigonometry
  Sin1 : Trigonometry
  Sin2 : Trigonometry
  Sum : Sum
  Sum{1..4} (4 alike) : Sum  Inputs=+-
  Va* : Outport
  Vb* : Outport  Port=2
  Vc* : Outport  Port=3
  wires:
  [sin_theta1] -> Product5/2
  [V_q] -> Product5/1
  [cos_theta1] -> Product4/2
  [V_d] -> Product4/1
  Product4/1 -> Sum4/1
  Product5/1 -> Sum4/2
  Sum4/1 -> Vc*/1
  [sin_theta2] -> Product3/2
  Sin2/1 -> [sin_theta2]
  Sin1/1 -> [sin_theta1]
  [V_q] -> Product3/1
  [cos_theta2] -> Product2/2
  [V_d] -> Product2/1
  Sum3/1 -> Vb*/1
  Product3/1 -> Sum3/2
  Product2/1 -> Sum3/1
  [sin_theta] -> Product1/2
  [V_q] -> Product1/1
  [cos_theta] -> Product/2
  [V_d] -> Product/1
  Product/1 -> Sum2/1
  Product1/1 -> Sum2/2
  Sum2/1 -> Va*/1
  Cos2/1 -> [cos_theta2]
  Cos1/1 -> [cos_theta1]
  Sum1/1 -> Cos2/1, Sin2/1
  Sum/1 -> Cos1/1, Sin1/1
  Constant/1 -> Sum/2, Sum1/2
  Sin/1 -> [sin_theta]
  Cos/1 -> [cos_theta]
  theta/1 -> Cos/1, Sin/1, Sum1/1, Sum/1
  V_d*/1 -> [V_d]
  V_q*/1 -> [V_q]

== system FOC_physical_2_Testing_mathmatical/Subsystem/Inverse Transformation/inverse Clark ==
  In1 : Inport
  In2 : Inport  Port=2
  Add : Sum
  Add1 : Sum
  Constant : Constant  Value=-1/2
  Constant1 : Constant  Value=sqrt(3)/2
  Constant2 : Constant  Value=-1/2
  Constant3 : Constant  Value=-sqrt(3)/2
  Product{,1..3} (4 alike) : Product
  Va : Outport
  Vb : Outport  Port=2
  Vc : Outport  Port=3
  wires:
  In1/1 -> Va/1, Product1/2, Product2/2
  In2/1 -> Product/1, Product3/2
  Add/1 -> Vb/1
  Product3/1 -> Add1/2
  Constant/1 -> Product1/1
  Constant2/1 -> Product2/1
  Product/1 -> Add/2
  Constant1/1 -> Product/2
  Product1/1 -> Add/1
  Product2/1 -> Add1/1
  Add1/1 -> Vc/1
  Constant3/1 -> Product3/1

== system FOC_physical_2_Testing_mathmatical/Subsystem/SVPWM/Subsystem ==
  Valpha : Inport
  Vbeta : Inport  Port=2
  Atan2 : Trigonometry  Operator=atan2
  Display : Display
  Display1 : Display
  Math Function : Math  Operator=square
  Math Function1 : Math  Operator=square
  Scope : Scope
  Sqrt1 : Sqrt
  Sum : Sum  Inputs=|++
  Vref : Outport
  angle : Outport  Port=2
  wires:
  Math Function1/1 -> Sum/2
  Valpha/1 -> Atan2/2, Math Function/1
  Vbeta/1 -> Atan2/1, Math Function1/1
  Sqrt1/1 -> Display/1, Vref/1, Scope/1
  Math Function/1 -> Sum/1
  Atan2/1 -> angle/1, Display1/1
  Sum/1 -> Sqrt1/1

== system FOC_physical_2_Testing_mathmatical/Subsystem/SVPWM/Subsystem1 ==
  Vref : Inport
  angle : Inport  Port=2
  Sector : Inport  Port=3
  Vdc : Inport  Port=4
  Add : Sum  Inputs=--+
  Constant4 : Constant  Value=T_period
  Constant5 : Constant  Value=pi/3
  Divide : Product  Inputs=*/
  Gain : Gain  Gain=(T_period)*sqrt(3)
  Product1 : Product
  Product2 : Product
  Sin : Trigonometry
  Sin1 : Trigonometry
  Subtract3 : Sum  Inputs=+-
  Theta dash : Subsystem
  T1 : Outport
  T2 : Outport  Port=2
  T0 : Outport  Port=3
  wires:
  Sector/1 -> Theta dash/1(Sector)
  Constant5/1 -> Subtract3/1
  angle/1 -> Theta dash/2(angle)
  Divide/1 -> Gain/1
  Vref/1 -> Divide/1
  Vdc/1 -> Divide/2
  Subtract3/1 -> Sin/1
  Gain/1 -> Product2/1, Product1/1
  Sin/1 -> Product1/2
  Sin1/1 -> Product2/2
  Product1/1 -> T1/1, Add/1
  Constant4/1 -> Add/3
  Product2/1 -> Add/2, T2/1
  Add/1 -> T0/1
  Theta dash/1(Theta dash) -> Sin1/1, Subtract3/2

== system FOC_physical_2_Testing_mathmatical/Subsystem/SVPWM/Subsystem2 ==
  T1 : Inport
  T2 : Inport  Port=2
  T0 : Inport  Port=3
  Sector definiton : Inport  Port=4
  Display : Display
  Fcn : Fcn  Expr=(T_period)-(u(3)/2)
  Fcn1 : Fcn  Expr=u(2)+(u(3)/2)
  Fcn2 : Fcn  Expr=u(3)/2
  Fcn3 : Fcn  Expr=u(1)+(u(3)/2)
  MATLAB Function : MATLAB Function  TreatAsAtomicUnit=on
  Mux : Mux  Inputs=3
  TS1 : Outport
  TS3 : Outport  Port=2
  TS5 : Outport  Port=3
  wires:
  MATLAB Function/1(TS1) -> TS1/1
  MATLAB Function/3(TS5) -> TS5/1
  MATLAB Function/2(TS3) -> TS3/1
  T1/1 -> Mux/1
  T2/1 -> Mux/2
  T0/1 -> Mux/3
  Mux/1 -> Display/1, Fcn1/1, Fcn/1, Fcn3/1, Fcn2/1
  Fcn/1 -> MATLAB Function/1(u)
  Fcn1/1 -> MATLAB Function/2(v)
  Fcn2/1 -> MATLAB Function/3(w)
  Fcn3/1 -> MATLAB Function/4(g)
  Sector definiton/1 -> MATLAB Function/5(S)

== system FOC_physical_2_Testing_mathmatical/Subsystem/SVPWM/Subsystem3 ==
  TS1 : Inport
  TS3 : Inport  Port=2
  TS5 : Inport  Port=3
  Carrier : Inport  Port=4
  Relational Operator : RelationalOperator  OutDataTypeStr=boolean  RndMeth=Simplest  InputSameDT=off
  Relational Operator1 : RelationalOperator  OutDataTypeStr=boolean  RndMeth=Simplest  InputSameDT=off
  Relational Operator2 : RelationalOperator  OutDataTypeStr=boolean  RndMeth=Simplest  InputSameDT=off
  Scope : Scope  NumInputPorts=3
  Pwm1 : Outport
  PWM3 : Outport  Port=2
  PWM5 : Outport  Port=3
  wires:
  TS1/1 -> Scope/1, Relational Operator/1
  TS3/1 -> Relational Operator1/1
  TS5/1 -> Relational Operator2/1
  Carrier/1 -> Scope/2, Relational Operator/2, Relational Operator1/2, Relational Operator2/2
  Relational Operator/1 -> Scope/3, Pwm1/1
  Relational Operator1/1 -> PWM3/1
  Relational Operator2/1 -> PWM5/1

== system FOC_physical_2_Testing_mathmatical/Subsystem/SVPWM/Subsystem4 ==
  TS1 : Inport
  TS3 : Inport  Port=2
  TS5 : Inport  Port=3
  NOT : Logic  Operator=NOT  IconShape=distinctive  AllPortsSameDT=off  OutDataTypeStr=boolean
  NOT1 : Logic  Operator=NOT  IconShape=distinctive  AllPortsSameDT=off  OutDataTypeStr=boolean
  NOT2 : Logic  Operator=NOT  IconShape=distinctive  AllPortsSameDT=off  OutDataTypeStr=boolean
  S1 : Outport
  S2 : Outport  Port=2
  S3 : Outport  Port=3
  S4 : Outport  Port=4
  S5 : Outport  Port=5
  S6 : Outport  Port=6
  wires:
  NOT2/1 -> S2/1
  TS5/1 -> NOT2/1, S5/1
  NOT1/1 -> S6/1
  TS3/1 -> S3/1, NOT1/1
  NOT/1 -> S4/1
  TS1/1 -> S1/1, NOT/1

== system FOC_physical_2_Testing_mathmatical/Subsystem/SVPWM/Valpha and Vbeta Clark Trans ==
  Va : Inport
  Vb : Inport  Port=2
  Vc : Inport  Port=3
  Add : Sum  Inputs=+++
  Add1 : Sum  Inputs=+-
  Gain : Gain  Gain=2/3
  Gain1 : Gain  Gain=-1/2
  Gain2 : Gain  Gain=-1/2
  Gain3 : Gain  Gain=2/3
  Gain5 : Gain  Gain=sqrt(3)/2
  Valpha : Outport
  Vbeta : Outport  Port=2
  wires:
  Gain1/1 -> Add/2
  Va/1 -> Add/1
  Add1/1 -> Gain5/1
  Gain2/1 -> Add/3
  Add/1 -> Gain/1
  Gain/1 -> Valpha/1
  Gain3/1 -> Vbeta/1
  Vb/1 -> Add1/1, Gain1/1
  Vc/1 -> Add1/2, Gain2/1
  Gain5/1 -> Gain3/1

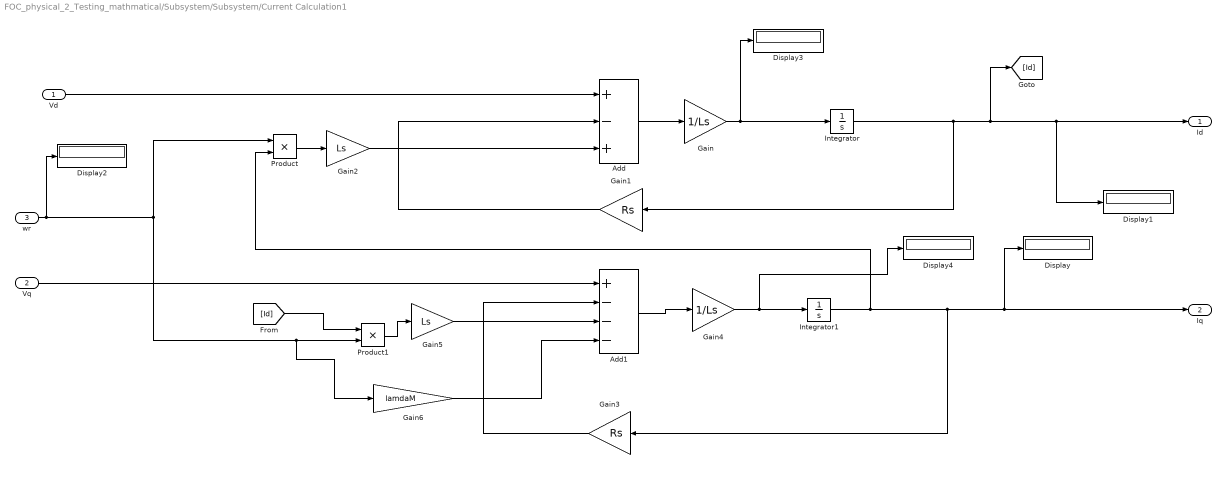
== system FOC_physical_2_Testing_mathmatical/Subsystem/Subsystem/Current Calculation1 ==
  Vd : Inport
  Vq : Inport  Port=2
  wr : Inport  Port=3
  Add : Sum  Inputs=+-+
  Add1 : Sum  Inputs=+---
  Display{,1..4} (5 alike) : Display
  Gain : Gain  Gain=1/Ls
  Gain1 : Gain  Gain=Rs
  Gain2 : Gain  Gain=Ls
  Gain3 : Gain  Gain=Rs
  Gain4 : Gain  Gain=1/Ls
  Gain5 : Gain  Gain=Ls
  Gain6 : Gain  Gain=lamdaM
  Integrator : Integrator
  Integrator1 : Integrator
  Product : Product
  Product1 : Product
  Id : Outport
  Iq : Outport  Port=2
  wires:
  Gain6/1 -> Add1/4
  Gain5/1 -> Add1/3
  Product1/1 -> Gain5/1
  [Id] -> Product1/1
  Gain3/1 -> Add1/2
  Integrator1/1 -> Gain3/1, Iq/1, Display/1, Product/2
  Gain4/1 -> Integrator1/1, Display4/1
  Add1/1 -> Gain4/1
  Vq/1 -> Add1/1
  Gain2/1 -> Add/3
  Product/1 -> Gain2/1
  wr/1 -> Display2/1, Product1/2, Gain6/1, Product/1
  Gain1/1 -> Add/2
  Integrator/1 -> Id/1, Display1/1, [Id], Gain1/1
  Gain/1 -> Display3/1, Integrator/1
  Add/1 -> Gain/1
  Vd/1 -> Add/1

== system FOC_physical_2_Testing_mathmatical/Subsystem/Subsystem/Park and Clark transformation1 ==
  Va : Inport
  Vb : Inport  Port=2
  Vc : Inport  Port=3
  Theta : Inport  Port=4
  Display{,1..7} (8 alike) : Display
  Subsystem : Subsystem
  Subsystem1 : Subsystem
  Vd : Outport
  Vq : Outport  Port=2
  wires:
  Theta/1 -> Subsystem1/1(Theta), Display7/1
  Subsystem1/2(Vq) -> Display1/1, Vq/1
  Subsystem1/1(Vd) -> Vd/1, Display/1
  Subsystem/2(Vbeta) -> Subsystem1/3(Vbeta), Display3/1
  Subsystem/1(Valpha) -> Subsystem1/2(Valpha), Display2/1
  Vc/1 -> Subsystem/3(In3), Display6/1
  Vb/1 -> Subsystem/2(In2), Display5/1
  Va/1 -> Subsystem/1(In1), Display4/1

== system FOC_physical_2_Testing_mathmatical/Subsystem/Subsystem/Speed1 ==
  Te : Inport
  TL : Inport  Port=2
  Add : Sum  Inputs=+---
  Constant : Constant  Value=2*pi
  Constant1 : Constant  Value=Tc
  Display : Display
  Display1 : Display
  Gain : Gain  Gain=1/J
  Gain1 : Gain  Gain=B
  Gain2 : Gain  Gain=P
  Integrator : Integrator
  Integrator2 : Integrator
  Rem : Math  Operator=rem
  wr : Outport
  Theta : Outport  Port=2
  wires:
  Constant1/1 -> Add/3
  Rem/1 -> Theta/1, Display/1
  Constant/1 -> Rem/2
  Integrator2/1 -> Rem/1
  Gain2/1 -> wr/1, Integrator2/1, Display1/1
  Gain1/1 -> Add/4
  Add/1 -> Gain/1
  TL/1 -> Add/2
  Gain/1 -> Integrator/1
  Te/1 -> Add/1
  Integrator/1 -> Gain1/1, Gain2/1

== system FOC_physical_2_Testing_mathmatical/Subsystem/Subsystem/Torque 1 ==
  Id : Inport
  Iq : Inport  Port=2
  Display : Display
  Display1 : Display
  Gain : Gain  Gain=lamdaM
  Gain1 : Gain  Gain=P
  Gain2 : Gain  Gain=3/2
  Gain3 : Gain
  Saturation : Saturate  UpperLimit=3.82  LowerLimit=-3.82
  Te : Outport
  wires:
  Gain3/1 -> Te/1
  Gain1/1 -> Gain2/1
  Gain2/1 -> Saturation/1
  Gain/1 -> Gain1/1
  Iq/1 -> Gain/1, Display1/1
  Saturation/1 -> Gain3/1, Display/1

== system FOC_physical_2_Testing_mathmatical/Subsystem/voltage limits by maintaining the same ration/Normal_Voltage ==
  Vq_ref_new : Inport
  Vd_ref_new : Inport  Port=2
  Action Port : ActionPort  ActionPortLabel=if(u1 <= 0)
  Data Type Conversion : DataTypeConversion  OutDataTypeStr=single  SaturateOnIntegerOverflow=off  RndMeth=Floor
  Data Type Conversion1 : DataTypeConversion  OutDataTypeStr=single  SaturateOnIntegerOverflow=off  RndMeth=Floor
  Vq_ref_1 : Outport
  Vd_ref_1 : Outport  Port=2
  wires:
  Vq_ref_new/1 -> Data Type Conversion/1
  Vd_ref_new/1 -> Data Type Conversion1/1
  Data Type Conversion/1 -> Vq_ref_1/1
  Data Type Conversion1/1 -> Vd_ref_1/1

== system FOC_physical_2_Testing_mathmatical/Subsystem/voltage limits by maintaining the same ration/Voltage_to_be_Limited ==
  Vq_ref_new : Inport
  Vd_ref_new : Inport  Port=2
  Action Port : ActionPort  ActionPortLabel=else
  Divide1 : Product  Inputs=*/  OutDataTypeStr=single
  Divide2 : Product  Inputs=/*  OutDataTypeStr=single
  Gain : Gain  Gain=sqrt(3)
  Gain1 : Gain  Gain=Vdc * ma
  Gain2 : Gain  Gain=Vdc * ma
  Square : Math  Operator=square  OutDataTypeStr=single
  Square Root : Sqrt  OutDataTypeStr=single  IntermediateResultsDataTypeStr=single
  Square1 : Math  Operator=square  OutDataTypeStr=single
  Sum : Sum  OutDataTypeStr=single  AccumDataTypeStr=single
  Vq_ref_2 : Outport
  Vd_ref_2 : Outport  Port=2
  wires:
  Vq_ref_new/1 -> Gain1/1, Square/1
  Sum/1 -> Square Root/1
  Vd_ref_new/1 -> Square1/1, Gain2/1
  Square1/1 -> Sum/2
  Square/1 -> Sum/1
  Divide1/1 -> Vq_ref_2/1
  Square Root/1 -> Gain/1
  Divide2/1 -> Vd_ref_2/1
  Gain/1 -> Divide2/1, Divide1/2
  Gain1/1 -> Divide1/1
  Gain2/1 -> Divide2/2

== system FOC_physical_2_Testing_mathmatical/Subsystem3/Inverse Transformation/Inverse Park  ==
  In1 : Inport
  In2 : Inport  Port=2
  In3 : Inport  Port=3
  Cos : Trigonometry  Operator=cos
  Cos1 : Trigonometry  Operator=cos
  Product{,1..3} (4 alike) : Product
  Sin : Trigonometry
  Sin1 : Trigonometry
  Subtract : Sum  Inputs=+-
  Subtract2 : Sum
  Valpha : Outport
  Vbeta : Outport  Port=2
  wires:
  Product3/1 -> Subtract2/1
  In3/1 -> Product2/2, Product1/2
  In1/1 -> Cos/1, [theta], Sin/1
  Subtract/1 -> Valpha/1  "Valpha"
  Product/1 -> Subtract/1
  Subtract2/1 -> Vbeta/1  "Vbeta"
  Product2/1 -> Subtract2/2
  Cos/1 -> Product/1
  Product1/1 -> Subtract/2
  [theta] -> Cos1/1
  In2/1 -> Product/2, Product3/1
  [theta] -> Sin1/1
  Sin/1 -> Product1/1
  Cos1/1 -> Product2/1
  Sin1/1 -> Product3/2

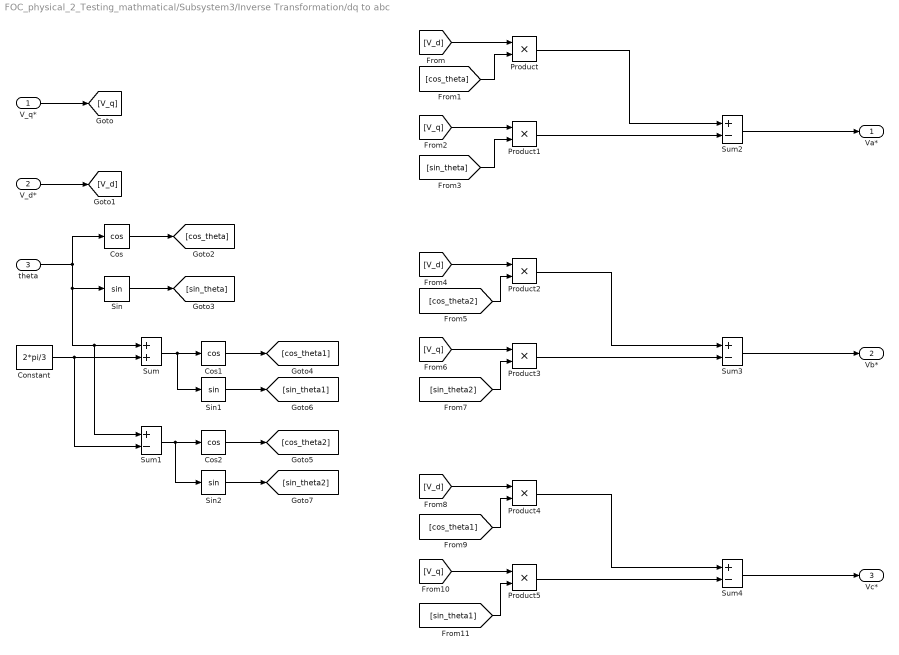
== system FOC_physical_2_Testing_mathmatical/Subsystem3/Inverse Transformation/dq to abc ==
  V_q* : Inport
  V_d* : Inport  Port=2
  theta : Inport  Port=3
  Constant : Constant  Value=2*pi/3
  Cos : Trigonometry  Operator=cos
  Cos1 : Trigonometry  Operator=cos
  Cos2 : Trigonometry  Operator=cos
  Product{,1..5} (6 alike) : Product
  Sin : Trigonometry
  Sin1 : Trigonometry
  Sin2 : Trigonometry
  Sum : Sum
  Sum{1..4} (4 alike) : Sum  Inputs=+-
  Va* : Outport
  Vb* : Outport  Port=2
  Vc* : Outport  Port=3
  wires:
  [sin_theta1] -> Product5/2
  [V_q] -> Product5/1
  [cos_theta1] -> Product4/2
  [V_d] -> Product4/1
  Product4/1 -> Sum4/1
  Product5/1 -> Sum4/2
  Sum4/1 -> Vc*/1
  [sin_theta2] -> Product3/2
  Sin2/1 -> [sin_theta2]
  Sin1/1 -> [sin_theta1]
  [V_q] -> Product3/1
  [cos_theta2] -> Product2/2
  [V_d] -> Product2/1
  Sum3/1 -> Vb*/1
  Product3/1 -> Sum3/2
  Product2/1 -> Sum3/1
  [sin_theta] -> Product1/2
  [V_q] -> Product1/1
  [cos_theta] -> Product/2
  [V_d] -> Product/1
  Product/1 -> Sum2/1
  Product1/1 -> Sum2/2
  Sum2/1 -> Va*/1
  Cos2/1 -> [cos_theta2]
  Cos1/1 -> [cos_theta1]
  Sum1/1 -> Cos2/1, Sin2/1
  Sum/1 -> Cos1/1, Sin1/1
  Constant/1 -> Sum/2, Sum1/2
  Sin/1 -> [sin_theta]
  Cos/1 -> [cos_theta]
  theta/1 -> Cos/1, Sin/1, Sum1/1, Sum/1
  V_d*/1 -> [V_d]
  V_q*/1 -> [V_q]

== system FOC_physical_2_Testing_mathmatical/Subsystem3/Inverse Transformation/inverse Clark ==
  In1 : Inport
  In2 : Inport  Port=2
  Add : Sum
  Add1 : Sum
  Constant : Constant  Value=-1/2
  Constant1 : Constant  Value=sqrt(3)/2
  Constant2 : Constant  Value=-1/2
  Constant3 : Constant  Value=-sqrt(3)/2
  Product{,1..3} (4 alike) : Product
  Va : Outport
  Vb : Outport  Port=2
  Vc : Outport  Port=3
  wires:
  In1/1 -> Va/1, Product1/2, Product2/2
  In2/1 -> Product/1, Product3/2
  Add/1 -> Vb/1
  Product3/1 -> Add1/2
  Constant/1 -> Product1/1
  Constant2/1 -> Product2/1
  Product/1 -> Add/2
  Constant1/1 -> Product/2
  Product1/1 -> Add/1
  Product2/1 -> Add1/1
  Add1/1 -> Vc/1
  Constant3/1 -> Product3/1

== system FOC_physical_2_Testing_mathmatical/Subsystem3/SVPWM/Subsystem ==
  Valpha : Inport
  Vbeta : Inport  Port=2
  Atan2 : Trigonometry  Operator=atan2
  Display : Display
  Display1 : Display
  Math Function : Math  Operator=square
  Math Function1 : Math  Operator=square
  Scope : Scope
  Sqrt1 : Sqrt
  Sum : Sum  Inputs=|++
  Vref : Outport
  angle : Outport  Port=2
  wires:
  Math Function1/1 -> Sum/2
  Valpha/1 -> Atan2/2, Math Function/1
  Vbeta/1 -> Atan2/1, Math Function1/1
  Sqrt1/1 -> Display/1, Vref/1, Scope/1
  Math Function/1 -> Sum/1
  Atan2/1 -> angle/1, Display1/1
  Sum/1 -> Sqrt1/1

== system FOC_physical_2_Testing_mathmatical/Subsystem3/SVPWM/Subsystem1 ==
  Vref : Inport
  angle : Inport  Port=2
  Sector : Inport  Port=3
  Vdc : Inport  Port=4
  Add : Sum  Inputs=--+
  Constant4 : Constant  Value=T_period
  Constant5 : Constant  Value=pi/3
  Divide : Product  Inputs=*/
  Gain : Gain  Gain=(T_period)*sqrt(3)
  Product1 : Product
  Product2 : Product
  Sin : Trigonometry
  Sin1 : Trigonometry
  Subtract3 : Sum  Inputs=+-
  Theta dash : Subsystem
  T1 : Outport
  T2 : Outport  Port=2
  T0 : Outport  Port=3
  wires:
  Sector/1 -> Theta dash/1(Sector)
  Constant5/1 -> Subtract3/1
  angle/1 -> Theta dash/2(angle)
  Divide/1 -> Gain/1
  Vref/1 -> Divide/1
  Vdc/1 -> Divide/2
  Subtract3/1 -> Sin/1
  Gain/1 -> Product2/1, Product1/1
  Sin/1 -> Product1/2
  Sin1/1 -> Product2/2
  Product1/1 -> T1/1, Add/1
  Constant4/1 -> Add/3
  Product2/1 -> Add/2, T2/1
  Add/1 -> T0/1
  Theta dash/1(Theta dash) -> Sin1/1, Subtract3/2

== system FOC_physical_2_Testing_mathmatical/Subsystem3/SVPWM/Subsystem2 ==
  T1 : Inport
  T2 : Inport  Port=2
  T0 : Inport  Port=3
  Sector definiton : Inport  Port=4
  Display : Display
  Fcn : Fcn  Expr=(T_period)-(u(3)/2)
  Fcn1 : Fcn  Expr=u(2)+(u(3)/2)
  Fcn2 : Fcn  Expr=u(3)/2
  Fcn3 : Fcn  Expr=u(1)+(u(3)/2)
  MATLAB Function : MATLAB Function  TreatAsAtomicUnit=on
  Mux : Mux  Inputs=3
  TS1 : Outport
  TS3 : Outport  Port=2
  TS5 : Outport  Port=3
  wires:
  MATLAB Function/1(TS1) -> TS1/1
  MATLAB Function/3(TS5) -> TS5/1
  MATLAB Function/2(TS3) -> TS3/1
  T1/1 -> Mux/1
  T2/1 -> Mux/2
  T0/1 -> Mux/3
  Mux/1 -> Display/1, Fcn1/1, Fcn/1, Fcn3/1, Fcn2/1
  Fcn/1 -> MATLAB Function/1(u)
  Fcn1/1 -> MATLAB Function/2(v)
  Fcn2/1 -> MATLAB Function/3(w)
  Fcn3/1 -> MATLAB Function/4(g)
  Sector definiton/1 -> MATLAB Function/5(S)

== system FOC_physical_2_Testing_mathmatical/Subsystem3/SVPWM/Subsystem3 ==
  TS1 : Inport
  TS3 : Inport  Port=2
  TS5 : Inport  Port=3
  Carrier : Inport  Port=4
  Relational Operator : RelationalOperator  OutDataTypeStr=boolean  RndMeth=Simplest  InputSameDT=off
  Relational Operator1 : RelationalOperator  OutDataTypeStr=boolean  RndMeth=Simplest  InputSameDT=off
  Relational Operator2 : RelationalOperator  OutDataTypeStr=boolean  RndMeth=Simplest  InputSameDT=off
  Scope : Scope  NumInputPorts=3
  Pwm1 : Outport
  PWM3 : Outport  Port=2
  PWM5 : Outport  Port=3
  wires:
  TS1/1 -> Scope/1, Relational Operator/1
  TS3/1 -> Relational Operator1/1
  TS5/1 -> Relational Operator2/1
  Carrier/1 -> Scope/2, Relational Operator/2, Relational Operator1/2, Relational Operator2/2
  Relational Operator/1 -> Scope/3, Pwm1/1
  Relational Operator1/1 -> PWM3/1
  Relational Operator2/1 -> PWM5/1

== system FOC_physical_2_Testing_mathmatical/Subsystem3/SVPWM/Subsystem4 ==
  TS1 : Inport
  TS3 : Inport  Port=2
  TS5 : Inport  Port=3
  NOT : Logic  Operator=NOT  IconShape=distinctive  AllPortsSameDT=off  OutDataTypeStr=boolean
  NOT1 : Logic  Operator=NOT  IconShape=distinctive  AllPortsSameDT=off  OutDataTypeStr=boolean
  NOT2 : Logic  Operator=NOT  IconShape=distinctive  AllPortsSameDT=off  OutDataTypeStr=boolean
  S1 : Outport
  S2 : Outport  Port=2
  S3 : Outport  Port=3
  S4 : Outport  Port=4
  S5 : Outport  Port=5
  S6 : Outport  Port=6
  wires:
  NOT2/1 -> S2/1
  TS5/1 -> NOT2/1, S5/1
  NOT1/1 -> S6/1
  TS3/1 -> S3/1, NOT1/1
  NOT/1 -> S4/1
  TS1/1 -> S1/1, NOT/1

== system FOC_physical_2_Testing_mathmatical/Subsystem3/SVPWM/Valpha and Vbeta Clark Trans ==
  Va : Inport
  Vb : Inport  Port=2
  Vc : Inport  Port=3
  Add : Sum  Inputs=+++
  Add1 : Sum  Inputs=+-
  Gain : Gain  Gain=2/3
  Gain1 : Gain  Gain=-1/2
  Gain2 : Gain  Gain=-1/2
  Gain3 : Gain  Gain=2/3
  Gain5 : Gain  Gain=sqrt(3)/2
  Valpha : Outport
  Vbeta : Outport  Port=2
  wires:
  Gain1/1 -> Add/2
  Va/1 -> Add/1
  Add1/1 -> Gain5/1
  Gain2/1 -> Add/3
  Add/1 -> Gain/1
  Gain/1 -> Valpha/1
  Gain3/1 -> Vbeta/1
  Vb/1 -> Add1/1, Gain1/1
  Vc/1 -> Add1/2, Gain2/1
  Gain5/1 -> Gain3/1

== system FOC_physical_2_Testing_mathmatical/Subsystem3/Subsystem/Current Calculation1 ==
  Vd : Inport
  Vq : Inport  Port=2
  wr : Inport  Port=3
  Add : Sum  Inputs=+-+
  Add1 : Sum  Inputs=+---
  Display{,1..4} (5 alike) : Display
  Gain : Gain  Gain=1/Ls
  Gain1 : Gain  Gain=Rs
  Gain2 : Gain  Gain=Ls
  Gain3 : Gain  Gain=Rs
  Gain4 : Gain  Gain=1/Ls
  Gain5 : Gain  Gain=Ls
  Gain6 : Gain  Gain=lamdaM
  Integrator : Integrator
  Integrator1 : Integrator
  Product : Product
  Product1 : Product
  Id : Outport
  Iq : Outport  Port=2
  wires:
  Gain6/1 -> Add1/4
  Gain5/1 -> Add1/3
  Product1/1 -> Gain5/1
  [Id] -> Product1/1
  Gain3/1 -> Add1/2
  Gain4/1 -> Integrator1/1, Display4/1
  Add1/1 -> Gain4/1
  Vq/1 -> Add1/1
  Gain2/1 -> Add/3
  Product/1 -> Gain2/1
  wr/1 -> Display2/1, Product1/2, Gain6/1, Product/1
  Gain1/1 -> Add/2
  Gain/1 -> Integrator/1, Display3/1
  Add/1 -> Gain/1
  Vd/1 -> Add/1
  Integrator/1 -> Id/1, Display1/1, [Id], Gain1/1
  Integrator1/1 -> Gain3/1, Iq/1, Display/1, Product/2

== system FOC_physical_2_Testing_mathmatical/Subsystem3/Subsystem/Park and Clark transformation1 ==
  Va : Inport
  Vb : Inport  Port=2
  Vc : Inport  Port=3
  Theta : Inport  Port=4
  Display{,1..7} (8 alike) : Display
  Subsystem : Subsystem
  Subsystem1 : Subsystem
  Vd : Outport
  Vq : Outport  Port=2
  wires:
  Theta/1 -> Subsystem1/1(Theta), Display7/1
  Subsystem1/2(Vq) -> Display1/1, Vq/1
  Subsystem1/1(Vd) -> Vd/1, Display/1
  Subsystem/2(Vbeta) -> Subsystem1/3(Vbeta), Display3/1
  Subsystem/1(Valpha) -> Subsystem1/2(Valpha), Display2/1
  Vc/1 -> Subsystem/3(In3), Display6/1
  Vb/1 -> Subsystem/2(In2), Display5/1
  Va/1 -> Subsystem/1(In1), Display4/1

== system FOC_physical_2_Testing_mathmatical/Subsystem3/Subsystem/Speed1 ==
  Te : Inport
  TL : Inport  Port=2
  Add : Sum  Inputs=+---
  Constant : Constant  Value=2*pi
  Constant1 : Constant  Value=Tc
  Display : Display
  Display1 : Display
  Gain : Gain  Gain=1/J
  Gain1 : Gain  Gain=B
  Gain2 : Gain  Gain=P
  Integrator : Integrator
  Integrator1 : Integrator
  Rem : Math  Operator=rem
  wr : Outport
  Theta : Outport  Port=2
  wires:
  Constant1/1 -> Add/3
  Rem/1 -> Theta/1, Display/1
  Constant/1 -> Rem/2
  Integrator/1 -> Rem/1
  Gain2/1 -> wr/1, Integrator/1, Display1/1
  Gain1/1 -> Add/4
  Add/1 -> Gain/1
  TL/1 -> Add/2
  Te/1 -> Add/1
  Gain/1 -> Integrator1/1
  Integrator1/1 -> Gain1/1, Gain2/1

== system FOC_physical_2_Testing_mathmatical/Subsystem3/Subsystem/Torque 1 ==
  Id : Inport
  Iq : Inport  Port=2
  Display : Display
  Display1 : Display
  Gain : Gain  Gain=lamdaM
  Gain1 : Gain  Gain=P
  Gain2 : Gain  Gain=3/2
  Gain3 : Gain
  Saturation : Saturate  UpperLimit=3.82  LowerLimit=-3.82
  Te : Outport
  wires:
  Gain3/1 -> Te/1
  Gain1/1 -> Gain2/1
  Gain2/1 -> Saturation/1
  Gain/1 -> Gain1/1
  Iq/1 -> Gain/1, Display1/1
  Saturation/1 -> Gain3/1, Display/1

== system FOC_physical_2_Testing_mathmatical/Subsystem3/voltage limits by maintaining the same ration/Normal_Voltage ==
  Vq_ref_new : Inport
  Vd_ref_new : Inport  Port=2
  Action Port : ActionPort  ActionPortLabel=if(u1 <= 0)
  Data Type Conversion : DataTypeConversion  OutDataTypeStr=single  SaturateOnIntegerOverflow=off  RndMeth=Floor
  Data Type Conversion1 : DataTypeConversion  OutDataTypeStr=single  SaturateOnIntegerOverflow=off  RndMeth=Floor
  Vq_ref_1 : Outport
  Vd_ref_1 : Outport  Port=2
  wires:
  Vq_ref_new/1 -> Data Type Conversion/1
  Vd_ref_new/1 -> Data Type Conversion1/1
  Data Type Conversion/1 -> Vq_ref_1/1
  Data Type Conversion1/1 -> Vd_ref_1/1
